simulink model "TestDynamicModel"  (R2022b)
settings: Solver=FixedStepAuto  StartTime=0.0  StopTime=40.0  FixedStep=simulator.TimeStep  RelTol=1e-3
undefined symbols (not defined in the file): simulator
settings Model: Creator=At  LastModifiedBy=ateay
settings SolverCC: ConcurrentTasks=on  AlgebraicLoopSolver=TrustRegion  InsertRTBMode=Never (minimum delay)
settings DataIOCC: ReturnWorkspaceOutputs=off
settings DebuggingCC: UnconnectedInputMsg=warning  UnconnectedOutputMsg=warning  UnconnectedLineMsg=warning  SFMachineParentedDataDiag=warning  ArithmeticOperatorsInVariantConditions=warning
settings ModelReferenceCC: EnableRefExpFcnMdlSchedulingChecks=on
settings SFSimCC: SimUseLocalCustomCode=off  CustomCodeUndefinedFunction=UseInterfaceOnly
settings RTWCC: RTWUseLocalCustomCode=off
settings CodeAppCC: StateflowObjectComments=on

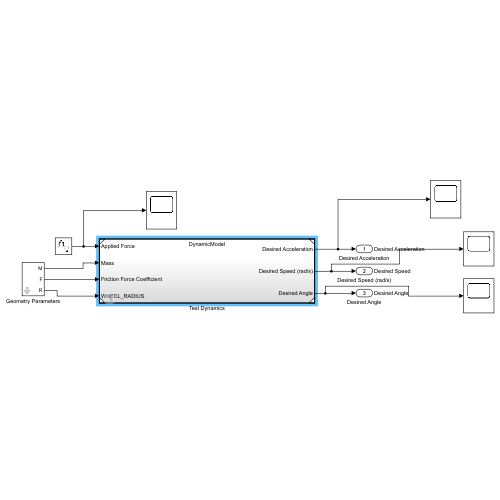
[thumbnail: Simulink's stored preview of the top-level diagram]
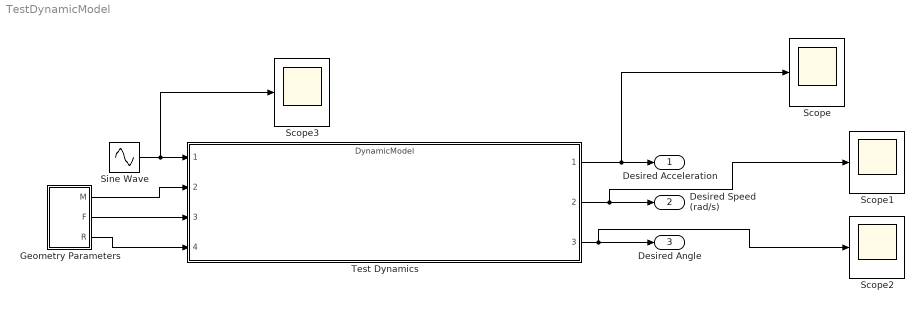
== system TestDynamicModel ==
  Geometry Parameters : Subsystem  mask{M=simulator.Sim.Dynamics.Mass, F=simulator.Sim.Dynamics.Friction.Coefficient, rR=simulator.Constants.WHEEL_RADIUS}
      mask prompts: M "Mass"; F "Friction"; rR "Radius"
      mask TypeOptions M: Mass/Value
      mask TypeOptions F: Friction/Value
      mask TypeOptions rR: rR/Value
  Scope{,1..3} (4 alike) : Scope
  Sine Wave : Sin  Amplitude=25  Frequency=4  SampleTime=1/2000
  "Test Dynamics " : ModelReference  ModelNameDialog=DynamicModel.slx  SimulationMode=Normal  ModelReferenceVersion=1.2
  Desired Acceleration : Outport  SignalName=Desired Acceleration
  Desired Speed (rad/s) : Outport  Port=2  SignalName=Desired Speed
  Desired Angle : Outport  Port=3  SignalName=Desired Angle
  wires:
  Geometry Parameters/3(R) -> "Test Dynamics "/4
  Geometry Parameters/2(F) -> "Test Dynamics "/3
  Geometry Parameters/1(M) -> "Test Dynamics "/2
  Sine Wave/1 -> Scope3/1, "Test Dynamics "/1
  "Test Dynamics "/3 -> Scope2/1, Desired Angle/1
  "Test Dynamics "/2 -> Scope1/1, Desired Speed (rad/s)/1
  "Test Dynamics "/1 -> Scope/1, Desired Acceleration/1

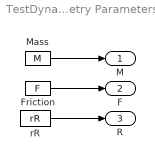
== system TestDynamicModel/Geometry Parameters ==
  Friction : Constant  Value=F
  Mass : Constant  Value=M
  rR : Constant  Value=rR
  M : Outport
  F : Outport  Port=2
  R : Outport  Port=3
  wires:
  Friction/1 -> F/1
  Mass/1 -> M/1
  rR/1 -> R/1
